simulink model "arith_enc_dec"  (R2023b)
settings: Solver=VariableStepAuto  StartTime=0.0  StopTime=10.0  RelTol=1e-3
settings SFSimCC: SimTargetLang=C++

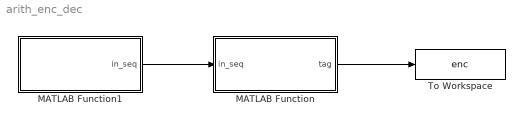
== system arith_enc_dec ==
  MATLAB Function : MATLAB Function  TreatAsAtomicUnit=on
  MATLAB Function1 : MATLAB Function  TreatAsAtomicUnit=on
  To Workspace : ToWorkspace  VariableName=enc  SaveFormat=Timeseries  SampleTime=-1
      settings: Save2DSignal=2-D array (concatenate along first dimension)
  wires:
  MATLAB Function/1(tag) -> To Workspace/1
  MATLAB Function1/1(in_seq) -> MATLAB Function/1(in_seq)

== matlab function arith_enc_dec/MATLAB Function1 ==
  data: in_seq output
function in_seq   = input_seq
    in = '1321';
    in_seq = double(char(in));
end

== matlab function arith_enc_dec/MATLAB Function ==
  data: in_seq input; tag output
function tag  = arith_enc(in_seq)
str=zeros(1,length(in_seq));
for r=1:length(in_seq)
    str(r)=char(in_seq(r));
end
str=char(str);
disp(['Input Sequence: ',str]);
len = length(str);

u = unique(str);
len_unique = length(u);

z = zeros(1,len_unique);
p = zeros(1,len_unique);

for i=1:len_unique
    z(i) = length(strfind(str,u(i)));
    p(i) = z(i)/len;
end

cpr = cumsum(p);

newcpr = [0 cpr];

interval = zeros(len_unique,2);

for i=1:len_unique    
    interval(i,1) = newcpr(i);
    interval(i,2) = cpr(i);
end

low=0;
high=1;

for i=1:len
    for j=1:len_unique
        if(str(i) == u(j))
            pos=j;
            j=j+1;
            range = high - low;
            high = low + (range*interval(pos,2));
            low = low + (range*interval(pos,1));
            i = i+1;
            break;
        end

    end
end
x=double(u);
u=x;
disp(['Probability: ']);
p
disp('The tag value is: ');
tag = low

%Decoding
pos=1;
str = zeros(1,length(in_seq));
k=1;
for i=1:len
    for j=1:len_unique
        if(tag >= interval(j,1) && tag < interval(j,2))
            pos = j;
            tag = (tag - interval(pos,1))/p(j);

            str(k) = u(pos);
            k=k+1;
            break;
        end

    end
end

disp(['Decoded String: ',str]);



end
